simulink model "diff_drive_sim"  (Simulink 10.0)
settings: Solver=VariableStepAuto  StartTime=0.0  StopTime=489.5  RelTol=1e-3
model workspace (MAT data in the model file):
  Kp : num (value not decoded)
values from neighbouring files (symbols this model uses):
  a = 4    [diff_drive.m]
  d = 3    [diff_drive.m]
  Kp = 5    [diff_drive.m]
  Kx = 15    [diff_drive.m]
  Ky = 15    [diff_drive.m]
  theta0 = pi/2    (= 1.57079632679)    [diff_drive.m]
  w = 0.1    [diff_drive.m]
  x0 = a    (= 4)    [diff_drive.m]
  y0 = 0    [diff_drive.m]
undefined symbols (not defined in the file or in its folder): gamma, Ktheta
settings Model: Creator=olivier  LastModifiedBy=johng
settings SolverCC: ZeroCrossAlgorithm=Adaptive
settings DataIOCC: SaveFormat=Dataset
settings OptimizationCC: LifeSpan=auto
settings DebuggingCC: UnderspecifiedInitializationDetection=Simplified  MergeDetectMultiDrivingBlocksExec=error  MaskedZcDiagnostic=none  SFUnexpectedBacktrackingDiag=error  SFNoUnconditionalDefaultTransitionDiag=error  SFExecutionAtInitializationDiag=warning
settings HardwareCC: ProdBitPerPointer=64  ProdBitPerSizeT=64  ProdBitPerPtrDiffT=64  ProdLargestAtomicFloat=Float  ProdIntDivRoundTo=Zero  ProdEndianess=LittleEndian  ProdWordSize=64  ProdHWDeviceType=Intel->x86-64 (Windows64)
settings ModelReferenceCC: PropagateSignalLabelsOutOfModel=on
settings SFSimCC: SimUseLocalCustomCode=on
settings RTWCC: RTWUseLocalCustomCode=on
settings CodeAppCC: StateflowObjectComments=off
settings GRTTargetCC: TargetLangStandard=C99 (ISO)  CombineOutputUpdateFcns=on  GRTInterface=off
settings ConfigComp: CovMetricSettings=dwe  CovHtmlReporting=off  CovSaveCumulativeToWorkspaceVar=off  CovSaveSingleToWorkspaceVar=off

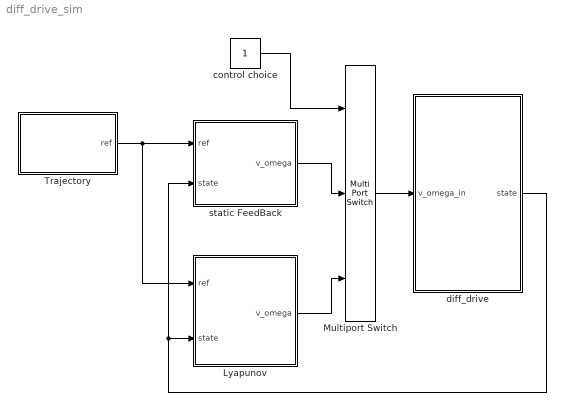
== system diff_drive_sim ==
  Lyapunov : Subsystem
  Multiport Switch : MultiPortSwitch  Inputs=2
  Trajectory : Subsystem  TreatAsAtomicUnit=on
  control choice : Constant
  diff_drive : Subsystem  mask{base=0.5, base_error=0, radius=0.2, radius_error=0, omega_max=80}
      mask prompts: base_error "Base error in percent"; radius_error "Radius error in percent"; omega_max "Wheel Max Velocity"
  static FeedBack : Subsystem
  wires:
  Trajectory/1(ref) -> Lyapunov/1(ref), static FeedBack/1(ref)
  static FeedBack/1(v_omega) -> Multiport Switch/2
  Multiport Switch/1 -> diff_drive/1(v_omega_in)
  control choice/1 -> Multiport Switch/1
  diff_drive/1(state) -> Lyapunov/2(state), static FeedBack/2(state)
  Lyapunov/1(v_omega) -> Multiport Switch/3

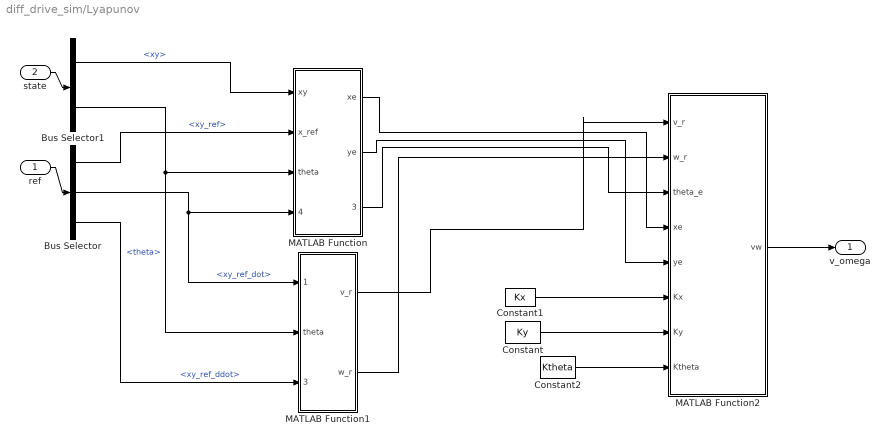
== system diff_drive_sim/Lyapunov ==
  ref : Inport
  state : Inport  Port=2
  Bus Selector : BusSelector  OutputSignals=xy_ref,xy_ref_dot,xy_ref_ddot
  Bus Selector1 : BusSelector  OutputSignals=xy,theta
  Constant : Constant  Value=Ky
  Constant1 : Constant  Value=Kx
  Constant2 : Constant  Value=Ktheta
  MATLAB Function : MATLAB Function  TreatAsAtomicUnit=on
  MATLAB Function1 : MATLAB Function  TreatAsAtomicUnit=on
  MATLAB Function2 : MATLAB Function  TreatAsAtomicUnit=on
  v_omega : Outport  VectorParamsAs1DForOutWhenUnconnected=off
  wires:
  MATLAB Function2/1(vw) -> v_omega/1
  ref/1 -> Bus Selector/1
  state/1 -> Bus Selector1/1
  Bus Selector/1 -> MATLAB Function/2(x_ref)  "<xy_ref>"
  Bus Selector/3 -> MATLAB Function1/3(x_ref_ddot)  "<xy_ref_ddot>"
  Bus Selector1/1 -> MATLAB Function/1(xy)  "<xy>"
  Bus Selector/2 -> MATLAB Function1/1(x_ref_dot), MATLAB Function/4(x_ref_dot)  "<xy_ref_dot>"
  Bus Selector1/2 -> MATLAB Function1/2(theta), MATLAB Function/3(theta)  "<theta>"
  MATLAB Function1/1(v_r) -> MATLAB Function2/1(v_r)
  MATLAB Function1/2(w_r) -> MATLAB Function2/2(w_r)
  MATLAB Function/1(xe) -> MATLAB Function2/4(xe)
  MATLAB Function/2(ye) -> MATLAB Function2/5(ye)
  MATLAB Function/3(theta_e) -> MATLAB Function2/3(theta_e)
  Constant1/1 -> MATLAB Function2/6(Kx)
  Constant/1 -> MATLAB Function2/7(Ky)
  Constant2/1 -> MATLAB Function2/8(Ktheta)

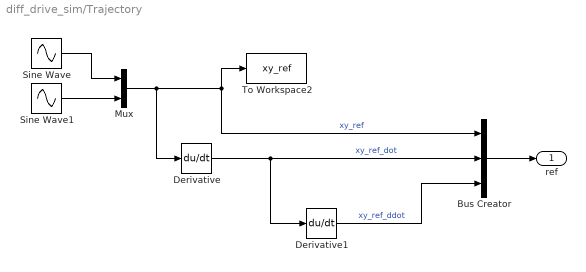
== system diff_drive_sim/Trajectory ==
  Bus Creator : BusCreator  Inputs=3
  Derivative : Derivative
  Derivative1 : Derivative
  Mux : Mux  Inputs=2
  Sine Wave : Sin  Amplitude=a  Frequency=w  Phase=pi/2  SampleTime=0
  Sine Wave1 : Sin  Amplitude=a  Frequency=w  SampleTime=0
  To Workspace2 : ToWorkspace  VariableName=xy_ref  SampleTime=-1
      settings: Save2DSignal=2-D array (concatenate along first dimension)
  ref : Outport  VectorParamsAs1DForOutWhenUnconnected=off
  wires:
  Bus Creator/1 -> ref/1
  Mux/1 -> Derivative/1, Bus Creator/1, To Workspace2/1  "xy_ref"
  Derivative/1 -> Bus Creator/2, Derivative1/1  "xy_ref_dot"
  Derivative1/1 -> Bus Creator/3  "xy_ref_ddot"
  Sine Wave1/1 -> Mux/2
  Sine Wave/1 -> Mux/1

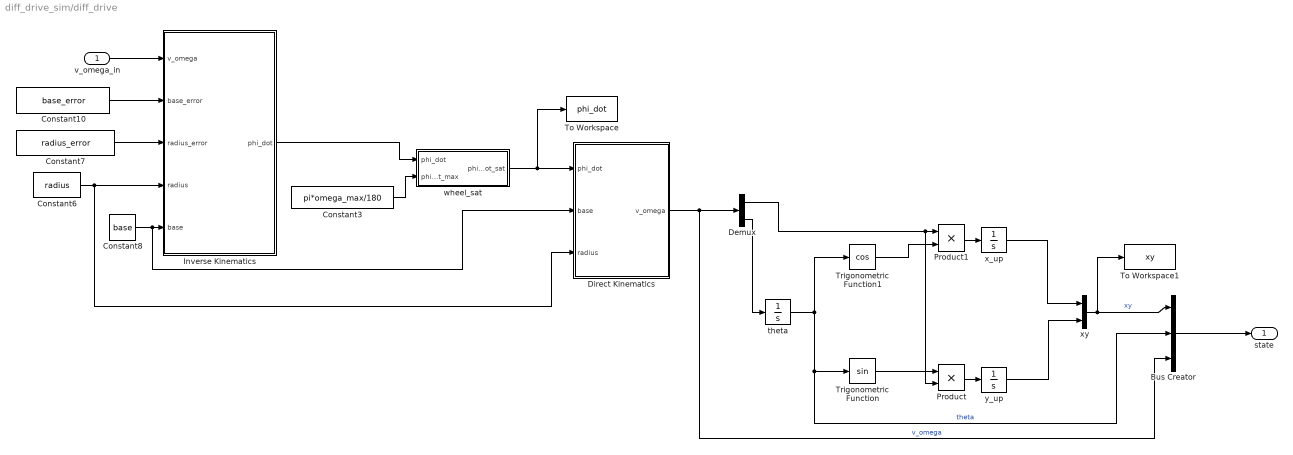
== system diff_drive_sim/diff_drive ==
  v_omega_in : Inport
  Bus Creator : BusCreator  Inputs=3
  Constant10 : Constant  Value=base_error
  Constant3 : Constant  Value=pi*omega_max/180
  Constant6 : Constant  Value=radius
  Constant7 : Constant  Value=radius_error
  Constant8 : Constant  Value=base
  Demux : Demux  Outputs=2
  Direct Kinematics : MATLAB Function  TreatAsAtomicUnit=on
  Inverse Kinematics : MATLAB Function  TreatAsAtomicUnit=on
  Product : Product
  Product1 : Product
  To Workspace : ToWorkspace  VariableName=phi_dot  SampleTime=-1
      settings: Save2DSignal=2-D array (concatenate along first dimension)
  To Workspace1 : ToWorkspace  VariableName=xy  SampleTime=-1
      settings: Save2DSignal=2-D array (concatenate along first dimension)
  Trigonometric Function : Trigonometry
  Trigonometric Function1 : Trigonometry  Operator=cos
  theta : Integrator  InitialCondition=theta0
  wheel_sat : Subsystem
  x_up : Integrator  InitialCondition=x0
  xy : Mux  Inputs=2
  y_up : Integrator  InitialCondition=y0
  state : Outport  VectorParamsAs1DForOutWhenUnconnected=off
  wires:
  theta/1 -> Trigonometric Function1/1, Trigonometric Function/1, Bus Creator/2  "theta"
  Trigonometric Function1/1 -> Product1/2
  Trigonometric Function/1 -> Product/1
  Product/1 -> y_up/1
  Product1/1 -> x_up/1
  x_up/1 -> xy/1
  Constant3/1 -> wheel_sat/2(phi_dot_max)
  Direct Kinematics/1(v_omega) -> Bus Creator/3, Demux/1  "v_omega"
  Demux/1 -> Product/2, Product1/1
  Demux/2 -> theta/1
  y_up/1 -> xy/2
  wheel_sat/1(phi_dot_sat) -> Direct Kinematics/1(phi_dot), To Workspace/1
  xy/1 -> Bus Creator/1, To Workspace1/1  "xy"
  Bus Creator/1 -> state/1
  Inverse Kinematics/1(phi_dot) -> wheel_sat/1(phi_dot)
  v_omega_in/1 -> Inverse Kinematics/1(v_omega)
  Constant10/1 -> Inverse Kinematics/2(base_error)
  Constant7/1 -> Inverse Kinematics/3(radius_error)
  Constant6/1 -> Inverse Kinematics/4(radius), Direct Kinematics/3(radius)
  Constant8/1 -> Direct Kinematics/2(base), Inverse Kinematics/5(base)

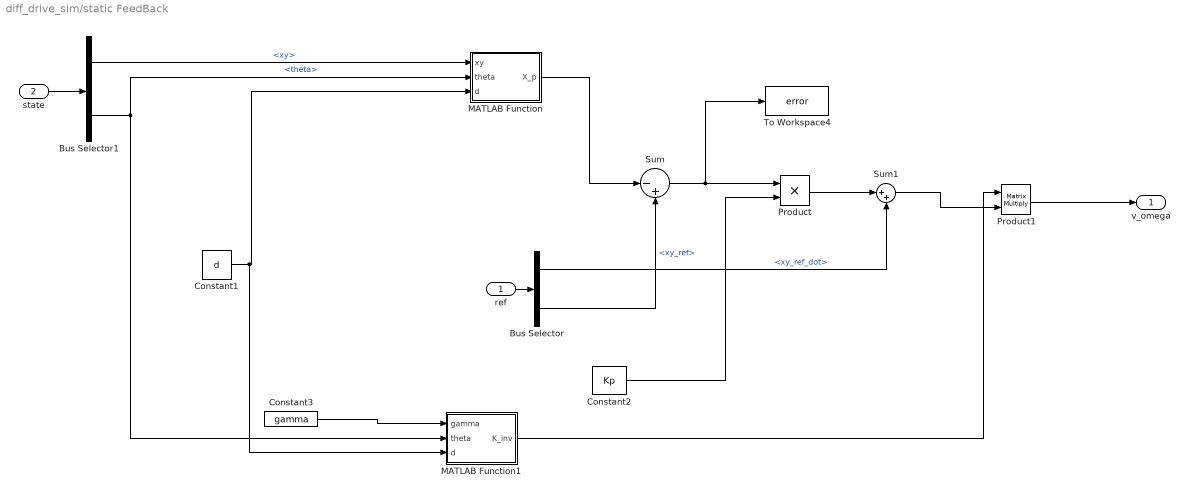
== system diff_drive_sim/static FeedBack ==
  ref : Inport
  state : Inport  Port=2
  Bus Selector : BusSelector  OutputSignals=xy_ref_dot,xy_ref
  Bus Selector1 : BusSelector  OutputSignals=xy,theta
  Constant1 : Constant  Value=d
  Constant2 : Constant  Value=Kp
  Constant3 : Constant  Value=gamma
  MATLAB Function : MATLAB Function  TreatAsAtomicUnit=on
  MATLAB Function1 : MATLAB Function  TreatAsAtomicUnit=on
  Product : Product
  Product1 : Product  Multiplication=Matrix(*)
  Sum : Sum  Inputs=|-+
  Sum1 : Sum  Inputs=|++
  To Workspace4 : ToWorkspace  VariableName=error  SampleTime=-1
      settings: Save2DSignal=2-D array (concatenate along first dimension)
  v_omega : Outport  VectorParamsAs1DForOutWhenUnconnected=off
  wires:
  ref/1 -> Bus Selector/1
  state/1 -> Bus Selector1/1
  Product1/1 -> v_omega/1
  MATLAB Function/1(X_p) -> Sum/1
  Constant2/1 -> Product/2
  Product/1 -> Sum1/1
  Sum1/1 -> Product1/2
  MATLAB Function1/1(K_inv) -> Product1/1
  Sum/1 -> To Workspace4/1, Product/1
  Bus Selector1/1 -> MATLAB Function/1(xy)  "<xy>"
  Bus Selector1/2 -> MATLAB Function1/2(theta), MATLAB Function/2(theta)  "<theta>"
  Constant1/1 -> MATLAB Function1/3(d), MATLAB Function/3(d)
  Constant3/1 -> MATLAB Function1/1(gamma)
  Bus Selector/1 -> Sum1/2  "<xy_ref_dot>"
  Bus Selector/2 -> Sum/2  "<xy_ref>"

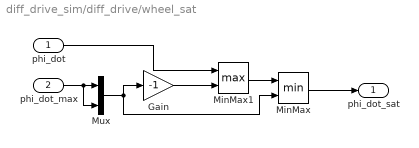
== system diff_drive_sim/diff_drive/wheel_sat ==
  phi_dot : Inport
  phi_dot_max : Inport  Port=2
  Gain : Gain  Gain=-1
  MinMax : MinMax  Inputs=2
  MinMax1 : MinMax  Function=max  Inputs=2
  Mux : Mux  Inputs=2
  phi_dot_sat : Outport  VectorParamsAs1DForOutWhenUnconnected=off
  wires:
  Gain/1 -> MinMax1/2
  MinMax/1 -> phi_dot_sat/1
  phi_dot_max/1 -> Mux/2, Mux/1
  phi_dot/1 -> MinMax1/1
  MinMax1/1 -> MinMax/1
  Mux/1 -> MinMax/2, Gain/1

== matlab function diff_drive/Inverse Kinematics ==
  data: v_omega input double; base_error input double; radius_error input double; radius input double; phi_dot output double; base input double
function phi_dot = ik(v_omega, base_error, radius_error, radius, base)

base = base * (1+base_error*0.01);
radius = radius * (1+radius_error*0.01);

phi_dot = [(v_omega(1)+base*v_omega(2))/radius; (v_omega(1)-base*v_omega(2))/radius];

== matlab function static FeedBack/MATLAB Function ==
  data: xy input double; X_p output double; theta input double; d input double
function X_p = fcn(xy,theta,d)

xp = xy(1) + d*cos(theta);
yp = xy(2) + d*sin(theta) ;

X_p = [xp;yp];
end

== matlab function static FeedBack/MATLAB Function1 ==
  data: gamma input double; K_inv output double; theta input double; d input double
function K_inv = K_inverse(gamma,theta , d)
K = [cos(theta),-d*sin(theta+gamma);sin(theta),d*cos(theta+gamma)];

K_inv = inv(K);
end

== matlab function diff_drive/Direct Kinematics ==
  data: phi_dot input double; v_omega output double; base input double; radius input double
function v_omega = dk(phi_dot, base, radius)

v_omega = [radius*(phi_dot(1)+phi_dot(2))/2; radius*(phi_dot(1)-phi_dot(2))/(2*base)];

== matlab function Lyapunov/MATLAB Function ==
  data: xy input double; xe output double; x_ref input double; theta input double; ye output double; theta_e output double; x_ref_dot input double
function [xe,ye,theta_e] = fcn(xy,x_ref,theta,x_ref_dot)
xe = cos (theta)*(x_ref(1) - xy(1)) + sin (theta)*( x_ref(2) - xy(2));
ye = -sin (theta)*(x_ref(1) - xy(1)) + cos( theta)*( x_ref(2) - xy(2));
theta_e = atan2(x_ref_dot(2),x_ref_dot(1))-theta ;
theta_e=theta_e-2*pi*floor((theta_e+pi)/(2*pi));
end

== matlab function Lyapunov/MATLAB Function1 ==
  data: x_ref_dot input double; v_r output double; theta input double; x_ref_ddot input double; w_r output double
function [v_r, w_r] = fcn2(x_ref_dot,theta,x_ref_ddot)
v_r = x_ref_dot(1)*cos(theta)+x_ref_dot(2)*sin(theta);
if v_r == 0
    w_r = 0;
else
   w_r = ((x_ref_dot(1)*x_ref_ddot(2))-(x_ref_ddot(1)*x_ref_dot(2)))/(v_r^2);

end

== matlab function Lyapunov/MATLAB Function2 ==
  data: v_r input double; vw output double; w_r input double; theta_e input double; xe input double; ye input double; Kx input double; Ky input double; Ktheta input double
function vw  = fcn3(v_r,w_r,theta_e,xe,ye,Kx,Ky,Ktheta)
v = v_r*cos(theta_e) + Kx*xe;
if theta_e == 0
    w = w_r+Ky*ye*v_r;
    vw = [v , w];
else
    w = (w_r+Ky*ye*v_r*(sin(theta_e)/theta_e))+Ktheta*theta_e;
vw = [v w];
end
